simulink model "convertidorboostbuenov2015"  (R2015a)
settings: Solver=ode45  StartTime=0.0  StopTime=2  RelTol=1e-3
values from neighbouring files (symbols this model uses):
  Al = [0 -Uss/L; Uss/C -1/(R*C)]    [sistemacontrolado.m]
  Bl = [-X2ss/L; X1ss/C]    [sistemacontrolado.m]
  CI = x(end,1:2)    [sistemacontrolado.m]
  Cl = [0 1]    [sistemacontrolado.m]
  Ki = k(1,3)    [sistemacontrolado.m]
  Kp = k(1,1:2)    [sistemacontrolado.m]
  ref = 240*sqrt(2)    [sistemacontrolado.m]
settings Model: CovModelRefEnable=off  Creator=blabala  LastModifiedBy=Administrador
settings DataIOCC: LimitDataPoints=off  SaveFormat=Dataset
settings HardwareCC: ProdBitPerPointer=64  ProdLargestAtomicFloat=Float  ProdIntDivRoundTo=Zero  ProdEndianess=LittleEndian  ProdHWDeviceType=Specified
settings ModelReferenceCC: PropagateSignalLabelsOutOfModel=on

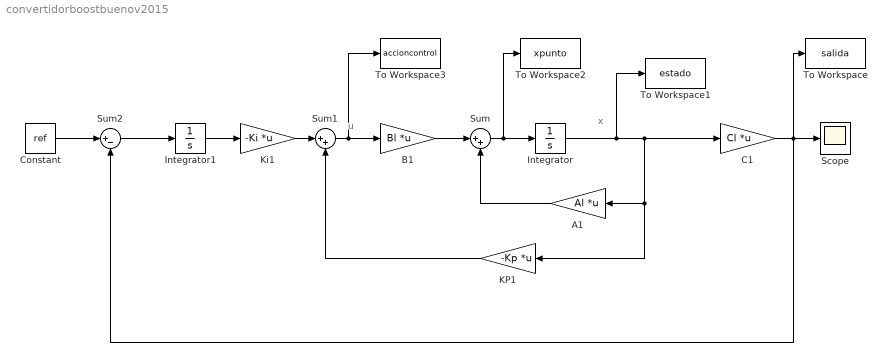
== system convertidorboostbuenov2015 ==
  note: x
  note: u
  A1 : Gain  Gain=Al  Multiplication=Matrix(K*u)
  B1 : Gain  Gain=Bl  Multiplication=Matrix(K*u)
  C1 : Gain  Gain=Cl  Multiplication=Matrix(K*u)
  Constant : Constant  Value=ref
  Integrator : Integrator  InitialCondition=CI
  Integrator1 : Integrator
  KP1 : Gain  Gain=-Kp  Multiplication=Matrix(K*u)
  Ki1 : Gain  Gain=-Ki  Multiplication=Matrix(K*u)
  Scope : Scope
      settings: YMin=-10  YMax=10
  Sum : Sum  Inputs=|++
  Sum1 : Sum  Inputs=|++
  Sum2 : Sum  Inputs=|+-
  To Workspace : ToWorkspace  VariableName=salida  SampleTime=-1
  To Workspace1 : ToWorkspace  VariableName=estado  SampleTime=-1
  To Workspace2 : ToWorkspace  VariableName=xpunto  SampleTime=-1
  To Workspace3 : ToWorkspace  VariableName=accioncontrol  SampleTime=-1
  wires:
  B1/1 -> Sum/1
  Sum/1 -> To Workspace2/1, Integrator/1
  C1/1 -> To Workspace/1, Sum2/2, Scope/1
  Integrator1/1 -> Ki1/1
  Ki1/1 -> Sum1/1
  Sum1/1 -> To Workspace3/1, B1/1
  Integrator/1 -> To Workspace1/1, C1/1, KP1/1, A1/1
  A1/1 -> Sum/2
  KP1/1 -> Sum1/2
  Constant/1 -> Sum2/1
  Sum2/1 -> Integrator1/1
